simulink model "Sim3e"  (R2016b)
settings: Solver=VariableStepAuto  StartTime=0.0  StopTime=total_time  RelTol=1e-3  EnableMultiTasking=on
values from neighbouring files (symbols this model uses):
  A = [-0.322 0.052 0.028 -1.12   0.002 ... (first row only)    [Copy_of_modelParms.m]    (also in modelParms.m)
  antiWindupBound = 0.05    [Copy_of_modelParms.m]    (also in modelParms.m)
  B = [0 0 0 0 10]'    [Copy_of_modelParms.m]    (also in modelParms.m)
  dist = deg2rad(2)    [Copy_of_modelParms.m]    (also in modelParms.m)
  g = 9.8    [Copy_of_modelParms.m]    (also in modelParms.m)
  Gamma_k = Gamma    [Copy_of_modelParms.m]
  H_k = C_kalman    [Copy_of_modelParms.m]
  k_d_phi = (2*zeta_phi*omega_n_phi - alpha_phi1)/alpha_phi2    [Copy_of_modelParms.m]    (also in modelParms.m)
  k_i_chi = omega_n_chi^2*V_g/g    [Copy_of_modelParms.m]    (also in modelParms.m)
  k_p_chi = 2*zeta_chi*omega_n_chi*V_g/g    [Copy_of_modelParms.m]    (also in modelParms.m)
  k_p_phi = delta_a_max/e_phi_max * sign(alpha_phi2)    [Copy_of_modelParms.m]    (also in modelParms.m)
  P_bar_0 = Q    [Copy_of_modelParms.m]
  Phi_k = Phi    [Copy_of_modelParms.m]
  Q_k = Q    [Copy_of_modelParms.m]
  R_k = R    [Copy_of_modelParms.m]
  V_g = 637 * 1000 / 3600    (= 176.944444444)    [Copy_of_modelParms.m]    (also in modelParms.m)
  x_bar_0 = [0, 0, 0, 0]'    [Copy_of_modelParms.m]
undefined symbols (not defined in the file or in its folder): Delta_k, n
settings Model: Creator=Alex  LastModifiedBy=Daniel
settings OptimizationCC: LifeSpan=inf
settings DebuggingCC: SFUnexpectedBacktrackingDiag=warning  SFNoUnconditionalDefaultTransitionDiag=warning  SFExecutionAtInitializationDiag=none
settings GRTTargetCC: TargetLangStandard=C89/C90 (ANSI)  GeneratePreprocessorConditionals=Disable all
settings ConfigComp: CovMetricSettings=dw  CovHtmlReporting=on  CovSaveCumulativeToWorkspaceVar=on  CovSaveSingleToWorkspaceVar=on  CovExternalEMLEnable=off

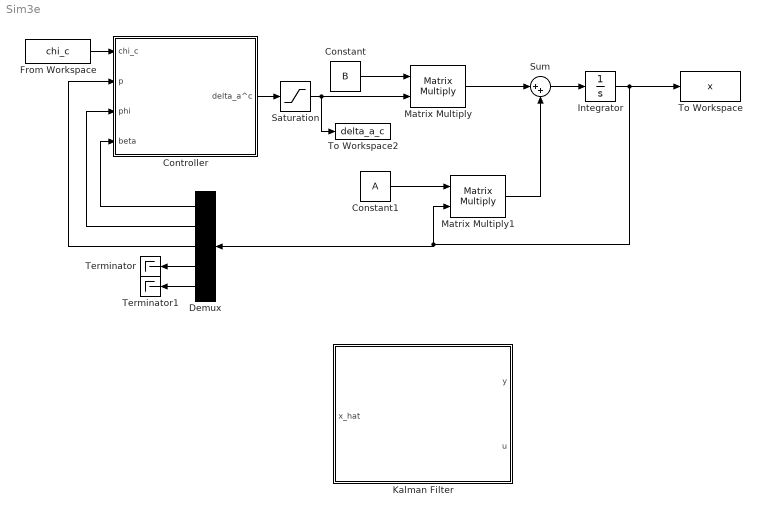
== system Sim3e ==
  Constant : Constant  Value=B
  Constant1 : Constant  Value=A
  Controller : Subsystem
  Demux : Demux  Outputs=5
  From Workspace : FromWorkspace  VariableName=chi_c  SampleTime=0
  Integrator : Integrator
  Kalman Filter : Subsystem
  Matrix Multiply : Product  Multiplication=Matrix(*)
  Matrix Multiply1 : Product  Multiplication=Matrix(*)
  Saturation : Saturate  UpperLimit=deg2rad(25)  LowerLimit=deg2rad(-25)
  Sum : Sum  Inputs=|++
  Terminator : Terminator
  Terminator1 : Terminator
  To Workspace : ToWorkspace  VariableName=x  SaveFormat=Timeseries  SampleTime=-1
  To Workspace2 : ToWorkspace  VariableName=delta_a_c  SaveFormat=Timeseries  SampleTime=-1
  wires:
  Controller/1(delta_a^c) -> Saturation/1
  Constant/1 -> Matrix Multiply/1
  Matrix Multiply/1 -> Sum/1
  Matrix Multiply1/1 -> Sum/2
  Constant1/1 -> Matrix Multiply1/1
  Sum/1 -> Integrator/1
  Demux/1 -> Controller/4(beta)
  Demux/2 -> Controller/3(phi)
  Demux/4 -> Terminator/1
  Demux/5 -> Terminator1/1
  Saturation/1 -> To Workspace2/1, Matrix Multiply/2
  Demux/3 -> Controller/2(p)
  From Workspace/1 -> Controller/1(chi_c)
  Integrator/1 -> Matrix Multiply1/2, Demux/1, To Workspace/1

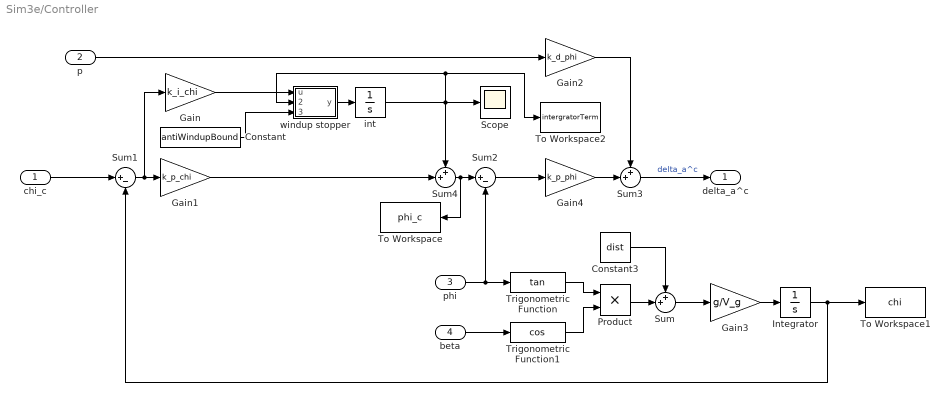
== system Sim3e/Controller ==
  chi_c : Inport
  p : Inport  Port=2
  phi : Inport  Port=3
  beta : Inport  Port=4
  Constant : Constant  Value=antiWindupBound
  Constant3 : Constant  Value=dist
  Gain : Gain  Gain=k_i_chi
  Gain1 : Gain  Gain=k_p_chi
  Gain2 : Gain  Gain=k_d_phi
  Gain3 : Gain  Gain=g/V_g
  Gain4 : Gain  Gain=k_p_phi
  Integrator : Integrator
  Product : Product
  Scope : Scope
  Sum : Sum  Inputs=++|
  Sum1 : Sum  Inputs=|+-
  Sum2 : Sum  Inputs=|+-
  Sum3 : Sum  Inputs=++|
  Sum4 : Sum  Inputs=++|
  To Workspace : ToWorkspace  VariableName=phi_c  SaveFormat=Timeseries  SampleTime=-1
  To Workspace1 : ToWorkspace  VariableName=chi  SaveFormat=Timeseries  SampleTime=-1
  To Workspace2 : ToWorkspace  VariableName=intergratorTerm  SaveFormat=Timeseries  SampleTime=-1
  Trigonometric Function : Trigonometry  Operator=tan
  Trigonometric Function1 : Trigonometry  Operator=cos
  int : Integrator
  windup stopper : MATLAB Function  TreatAsAtomicUnit=on
  delta_a^c : Outport
  wires:
  Sum3/1 -> delta_a^c/1  "delta_a^c"
  Gain3/1 -> Integrator/1
  Trigonometric Function1/1 -> Product/2
  Trigonometric Function/1 -> Product/1
  beta/1 -> Trigonometric Function1/1
  Gain4/1 -> Sum3/2
  Sum4/1 -> To Workspace/1, Sum2/1
  p/1 -> Gain2/1
  chi_c/1 -> Sum1/1
  Gain1/1 -> Sum4/2
  Sum1/1 -> Gain1/1, Gain/1
  Sum2/1 -> Gain4/1
  Gain2/1 -> Sum3/1
  int/1 -> Scope/1, windup stopper/2(compare), To Workspace2/1, Sum4/1
  phi/1 -> Sum2/2, Trigonometric Function/1
  Integrator/1 -> Sum1/2, To Workspace1/1
  Gain/1 -> windup stopper/1(u)
  windup stopper/1(y) -> int/1
  Constant/1 -> windup stopper/3(antiWindupBound)
  Product/1 -> Sum/2
  Constant3/1 -> Sum/1
  Sum/1 -> Gain3/1

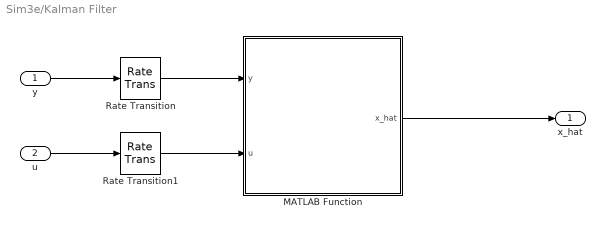
== system Sim3e/Kalman Filter ==
  y : Inport
  u : Inport  Port=2
  MATLAB Function : MATLAB Function  TreatAsAtomicUnit=on
  Rate Transition : RateTransition
  Rate Transition1 : RateTransition
  x_hat : Outport
  wires:
  Rate Transition1/1 -> MATLAB Function/2(u)
  Rate Transition/1 -> MATLAB Function/1(y)
  u/1 -> Rate Transition1/1
  y/1 -> Rate Transition/1
  MATLAB Function/1(x_hat) -> x_hat/1

== matlab function Sim3e/Controller/windup stopper ==
  data: u input; y output; compare input; antiWindupBound input
function y = fcn(u,compare, antiWindupBound)
%#codegen
if((abs(compare) >= antiWindupBound) && sign(u) == sign(compare))
    y = 0;
else
    y=u;
end

== matlab function Sim3e/Kalman Filter/MATLAB Function ==
  data: y input; u input; x_hat output; x_bar_0 parameter; Phi_k parameter; Delta_k parameter; Gamma_k parameter; H_k parameter; Q_k parameter; R_k parameter; n parameter; P_bar_0 parameter
function x_hat = fcn(y, u, x_bar_0, Phi_k, Delta_k, Gamma_k, H_k, Q_k, R_k, n, P_bar_0)

persistent P_hat_k;                                                 % Error covariance
persistent P_bar_k;                                                 % Error covariance prediction
persistent K_k;                                                     % Kalman gain matrix
persistent x_bar_k;                                                 % State prediction
persistent k;                                                       % Time step

if(isempty(k))
    % Initialize
    k = 0;                                                          % Time step zero
    P_bar_k = P_bar_0;                                                % Initial error covariance
    x_bar_k = x_bar_0;                                              % Initial state estimate
else
    % Iterate
    k = k + 1;                                                      % Time step
end

% Correction
K_k = P_bar_k*(H_k')/(H_k*P_k(H_k')+R_k);                           % Kalman gain matrix
x_hat_k = x_bar_k + K_k*(y + H_k*x_bar_k);                          % State error update
P_hat_k = (eye(n) - K_k*H_k)*P_bar_k*((I-K_k*H_k)') + K_k*R_k*K_k;  % Error covariance update

% Prediction
x_bar_k_pluss_one = Phi_k*x_hat_k + Delta_k*u;                      % State prediction
P_bar_k_pluss_one = Phi_k*P_hat_k*(Phi_k') + Gamma_k*Q_k*(Gamma_k');% Error covariance prediction

% Propagation
x_bar_k = x_bar_k_pluss_one;                                        % State estimate propagation
P_bar_k = P_bar_k_pluss_one;                                        % Error covariance propagation

% State estimate output
x_hat = x_hat_k;
